simulink model "lab2sim"  (R2022a)
settings: Solver=ode45  StartTime=0.0  StopTime=10  RelTol=1e-6  AbsTol=1e-6
undefined symbols (not defined in the file or in its folder): DiscIntNeverNeededParam
settings Model: Creator=ivans2  LastModifiedBy=ivans2
settings SolverCC: AutoScaleAbsTol=off

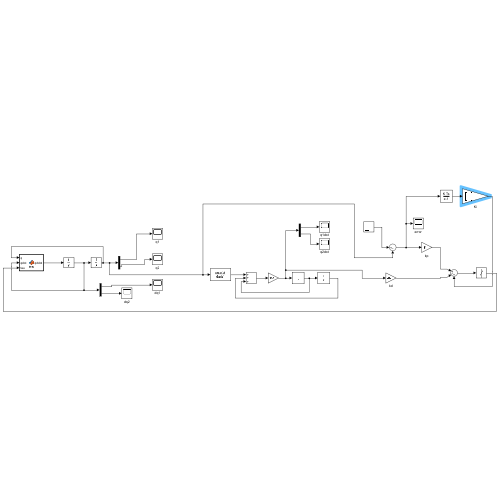
[thumbnail: Simulink's stored preview of the top-level diagram]
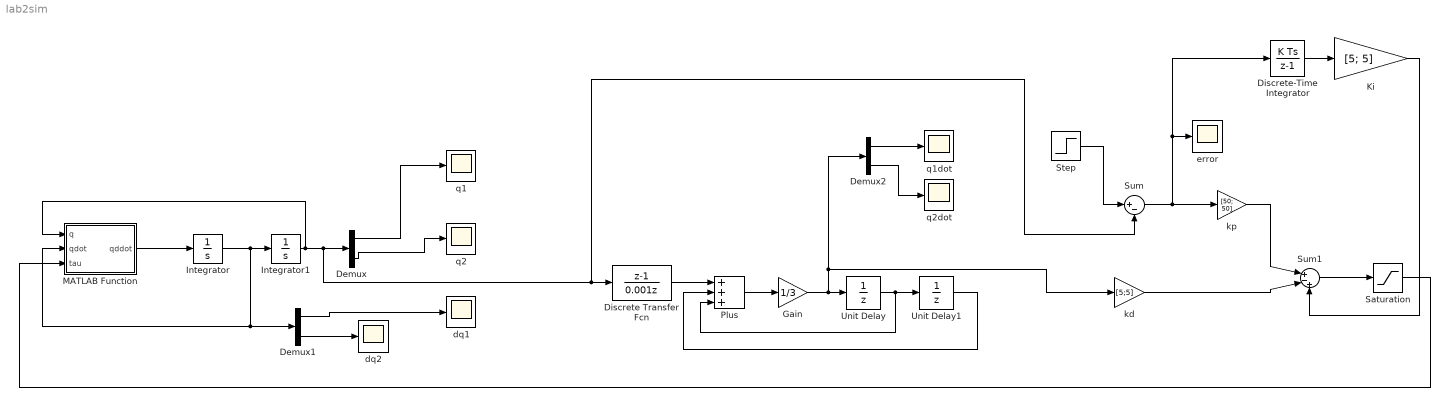
== system lab2sim ==
  Demux : Demux  Outputs=2
  Demux1 : Demux  Outputs=2
  Demux2 : Demux  Outputs=2
  Discrete Transfer Fcn : DiscreteTransferFcn  Numerator=[1 -1]  Denominator=[0.001 0]  SampleTime=0.001
  Discrete-Time Integrator : DiscreteIntegrator  SampleTime=0.001  ICPrevOutput=DiscIntNeverNeededParam  ICPrevScaledInput=DiscIntNeverNeededParam
  Gain : Gain  Gain=1/3
  Integrator : Integrator  InitialCondition=[0;0]
  Integrator1 : Integrator  InitialCondition=[0;0]
  Ki : Gain  Gain=[5; 5]
  MATLAB Function : MATLAB Function  TreatAsAtomicUnit=on
  Plus : Sum  Inputs=+++
  Saturation : Saturate  UpperLimit=5  LowerLimit=-5
  Step : Step  Time=0  After=[.25; .25]  SampleTime=0
  Sum : Sum  Inputs=|+-
  Sum1 : Sum  Inputs=|+-+
  Unit Delay : UnitDelay  SampleTime=0.001  HasFrameUpgradeWarning=on
  Unit Delay1 : UnitDelay  SampleTime=0.001  HasFrameUpgradeWarning=on
  dq1 : Scope
  dq2 : Scope
  error : Scope
  kd : Gain  Gain=[5;5]
  kp : Gain  Gain=[50; 50]
  q1 : Scope
  q1dot : Scope
  q2 : Scope
  q2dot : Scope
  wires:
  MATLAB Function/1(qddot) -> Integrator/1
  Integrator/1 -> MATLAB Function/2(qdot), Demux1/1, Integrator1/1
  Integrator1/1 -> MATLAB Function/1(q), Sum/2, Discrete Transfer Fcn/1, Demux/1
  Demux/1 -> q1/1
  Demux/2 -> q2/1
  Demux1/2 -> dq2/1
  Demux1/1 -> dq1/1
  Discrete Transfer Fcn/1 -> Plus/1
  Unit Delay/1 -> Plus/3, Unit Delay1/1
  Gain/1 -> Demux2/1, kd/1, Unit Delay/1
  Plus/1 -> Gain/1
  Unit Delay1/1 -> Plus/2
  Demux2/1 -> q1dot/1
  kd/1 -> Sum1/2
  kp/1 -> Sum1/1
  Step/1 -> Sum/1
  Sum/1 -> Discrete-Time Integrator/1, error/1, kp/1
  Saturation/1 -> MATLAB Function/3(tau)
  Sum1/1 -> Saturation/1
  Demux2/2 -> q2dot/1
  Discrete-Time Integrator/1 -> Ki/1
  Ki/1 -> Sum1/3

== matlab function lab2sim/MATLAB Function ==
  data: q input; qddot output; qdot input; tau input
function qddot = fcn(q, qdot, tau)
th2m = q(1);
th3m = q(2);
th2mdot = qdot(1);
th3mdot = qdot(2);
g = 9.8;


%%p1 = pars(1);
%%p2 = pars(2);
%%p3 = pars(3);
%%p4 = pars(4);
%%p5 = pars(5);

p1 = 0.0300;
p2 = 0.0128;
p3 = 0.0076;
p4 = 0.0753;
p5 = 0.0298;

D = [
[p1 -p3*sin(th3m - th2m)];
[-p3*sin(th3m - th2m) p2];
];

C = [
[0 -p3*cos(th3m - th2m)*th3mdot];
[p3*cos(th3m - th2m)*th2mdot 0];
];

G = [
[-p4*g*sin(th2m)];
[-p5*g*cos(th3m)];
];

qddot = zeros(2, 1);
qddot = inv(D)*(tau - C*qdot - G);
end
